simulink model "Tutorial1_DiscreteFilter"  (Simulink 9.1)
settings: Solver=FixedStepAuto  StartTime=0.0  StopTime=10.0  FixedStep=0.01  RelTol=1e-3
libraries: WBToolboxLibrary x2
settings Model: SuppressorTable=22 serialization::archive 11 0 6 0 0 0 1 0  Creator=dferigo  LastModifiedBy=dferigo
settings DataIOCC: SaveFormat=Dataset
settings OptimizationCC: LifeSpan=auto
settings DebuggingCC: UnderspecifiedInitializationDetection=Simplified  MergeDetectMultiDrivingBlocksExec=error  SFUnexpectedBacktrackingDiag=error  SFNoUnconditionalDefaultTransitionDiag=error  SFExecutionAtInitializationDiag=warning
settings HardwareCC: ProdBitPerPointer=64  ProdBitPerSizeT=64  ProdBitPerPtrDiffT=64  ProdLargestAtomicFloat=Float  ProdIntDivRoundTo=Zero  ProdEndianess=LittleEndian  ProdWordSize=64  ProdHWDeviceType=Intel->x86-64 (Windows64)
settings ModelReferenceCC: PropagateSignalLabelsOutOfModel=on
settings CodeAppCC: StateflowObjectComments=off
settings GRTTargetCC: TargetLangStandard=C99 (ISO)  CombineOutputUpdateFcns=on  GRTInterface=off
settings ConfigComp: CovMetricSettings=dwe  CovHtmlReporting=off  CovSaveCumulativeToWorkspaceVar=off  CovSaveSingleToWorkspaceVar=off  CovExternalEMLEnable=on

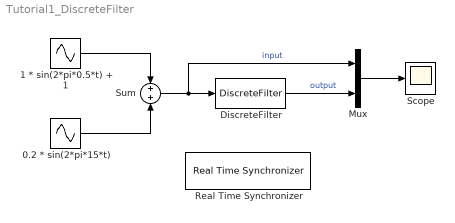
== system Tutorial1_DiscreteFilter ==
  0.2 * sin(2*pi*15*t) : Sin  Amplitude=0.2  Frequency=2*pi*15  SampleTime=0
  1 * sin(2*pi*0.5*t) + 1 : Sin  Bias=1  Frequency=2*pi*0.5  SampleTime=0
  DiscreteFilter : WBToolboxLibrary/Utilities/DiscreteFilter  filterType=FirstOrderLowPassFilter  numCoeffs=[0]  denCoeffs=[0]  Fc=2  Ts=0.01  orderMedianFilter=0  initStatus=off  y0=[0]  u0=[0]
      settings: SourceProductName=WholeBodyToolbox
  Mux : Mux  Inputs=2
  Real Time Synchronizer : WBToolboxLibrary/Utilities/Real Time Synchronizer  period=0.01
      settings: SourceProductName=WholeBodyToolbox
  Scope : Scope
  Sum : Sum  Inputs=+|+
  wires:
  1 * sin(2*pi*0.5*t) + 1/1 -> Sum/1
  0.2 * sin(2*pi*15*t)/1 -> Sum/2
  Sum/1 -> Mux/1, DiscreteFilter/1  "input"
  DiscreteFilter/1 -> Mux/2  "output"
  Mux/1 -> Scope/1
